simulink model "Exp9"  (R2018a)
settings: Solver=VariableStepAuto  StartTime=0.0  StopTime=0.2  RelTol=1e-3
libraries: powerlib x21
settings Model: Creator=Asus  LastModifiedBy=Asus

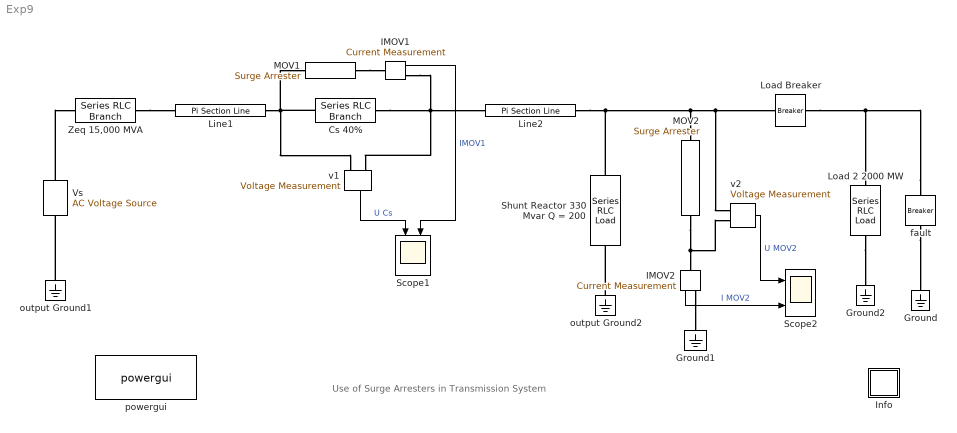
== system Exp9 ==
  note: Use of Surge Arresters in Transmission System
  Cs 40% : powerlib/Elements/Series RLC Branch  LConnTagsString=__new0  RConnTagsString=__new0  BranchType=C  Resistance=[]  Inductance=[]  SetiL0=off  InitialCurrent=0  Capacitance=101.4e-6  Setx0=off  InitialVoltage=0  Measurements=None
  Ground : powerlib/Elements/Ground  LConnTagsString=a
  Ground1 : powerlib/Elements/Ground  LConnTagsString=a
  Ground2 : powerlib/Elements/Ground  LConnTagsString=a
  IMOV1 : powerlib/Measurements/Current Measurement  Tag=PoWeRsYsTeMmEaSuReMeNt  PhasorSimulation=off  OutputType=Magnitude  PSBequivalent=0
  IMOV2 : powerlib/Measurements/Current Measurement  Tag=PoWeRsYsTeMmEaSuReMeNt  PhasorSimulation=off  OutputType=Magnitude  PSBequivalent=0
  Info : Subsystem
      settings: OpenFcn=showdemo(bdroot(gcb))
      mask Display: disp('?')
  Line1 : powerlib/Elements/Pi Section Line  LConnTagsString=__new0  RConnTagsString=__new0  Frequency=60  Resistance=0.011  Inductance=0.8674e-3  Capacitance=13.41e-9  Length=100  PiSections=2  Measurements=None
      settings: AttributesFormatString=\n  SourceProductName=Simscape Power Systems  SourceProductBaseCode=PS
  Line2 : powerlib/Elements/Pi Section Line  LConnTagsString=__new0  RConnTagsString=__new0  Frequency=60  Resistance=0.011  Inductance=0.8674e-3  Capacitance=13.41e-9  Length=100  PiSections=2  Measurements=None
      settings: AttributesFormatString=\n  SourceProductName=Simscape Power Systems  SourceProductBaseCode=PS
  Load 2 2000 MW : powerlib/Elements/Series RLC Load  LConnTagsString=a  RConnTagsString=__new0  NominalVoltage=735e3/sqrt(3)  NominalFrequency=60  ActivePower=2000e6/3  InductivePower=0  CapacitivePower=0  Setx0=off  InitialVoltage=0  SetiL0=off  InitialCurrent=0  Measurements=None  LoadType=constant Z
  Load Breaker : powerlib/Elements/Breaker  InitialState=1  SwitchingTimes=[ 100e-3]  External=off  BreakerResistance=0.1  SnubberResistance=inf  SnubberCapacitance=0  Measurements=None  MoreParameters=off  NoBreakLoop=off
      settings: AttributesFormatString=\n  SourceProductName=Simscape Power Systems
  MOV1 : powerlib/Elements/Surge Arrester  ProtectionVoltage=185e3  Columns=30  ReferenceCurrent=500  Segment1=[.955 50]  Segment2=[1.0 25]  Segment3=[.9915 16.5]  Measurements=None  BreakLoop=off
      settings: AttributesFormatString=\n  SourceProductName=Simscape Power Systems  SourceProductBaseCode=PS
  MOV2 : powerlib/Elements/Surge Arrester  ProtectionVoltage=1081e3  Columns=2  ReferenceCurrent=500  Segment1=[.955 50]  Segment2=[1.0 25]  Segment3=[.9915 16.5]  Measurements=None  BreakLoop=off
      settings: AttributesFormatString=\n  SourceProductName=Simscape Power Systems  SourceProductBaseCode=PS
  Scope1 : Scope  NumInputPorts=2
  Scope2 : Scope  NumInputPorts=2
  Shunt Reactor 330 Mvar Q = 200 : powerlib/Elements/Series RLC Load  LConnTagsString=a  RConnTagsString=__new0  NominalVoltage=735e3/sqrt(3)  NominalFrequency=60  ActivePower=330e6/3/200  InductivePower=330e6/3  CapacitivePower=0  Setx0=off  InitialVoltage=0  SetiL0=off  InitialCurrent=0  Measurements=None  LoadType=constant Z
  Vs : powerlib/Electrical Sources/AC Voltage Source  Description=source block  Amplitude=735e3/sqrt(3)*sqrt(2)  Phase=0  Frequency=60  SampleTime=0  Measurements=None  BusType=swing  Pref=10e3  Qref=0  Qmin=-inf  Qmax=+inf
      settings: AttributesFormatString=\n
  Zeq 15,000 MVA : powerlib/Elements/Series RLC Branch  LConnTagsString=__new0  RConnTagsString=__new0  BranchType=RL  Resistance=3.6  Inductance=95.5e-3  SetiL0=off  InitialCurrent=0  Capacitance=[]  Setx0=off  InitialVoltage=0  Measurements=None
  fault : powerlib/Elements/Breaker  InitialState=0  SwitchingTimes=[ 30e-3 300e-3]  External=off  BreakerResistance=1  SnubberResistance=inf  SnubberCapacitance=0  Measurements=None  MoreParameters=off  NoBreakLoop=off
      settings: AttributesFormatString=\n  SourceProductName=Simscape Power Systems
  output Ground1 : powerlib/Elements/Ground  LConnTagsString=a
  output Ground2 : powerlib/Elements/Ground  LConnTagsString=a
  powergui : powerlib/powergui  Priority=2  SimulationMode=Continuous  SampleTime=50e-6  frequency=60  Iterations=50  frequencyindice=60  Pbase=100e6  ErrMax=1e-4  UnitsV=kV  UnitsW=MW  buscounter=0  FunctionMessages=off  echomessages=off  EnableUseOfTLC=off  CurrentSourceSwitches=off  DisableSnubberDevices=off  DisableRonSwitches=off  DisableVfSwitches=off  DisplayEquations=off  SolverType=Tustin/Backward Euler (TBE)  Interpol=off  ExternalGateDelay=off  methode=off  Ts=100  x0status=blocks  SPID=on  SwTol=0  HookPort=off  RestoreLinks=warning  ResistiveCurrentMeasurement=off  Frange=logspace(0,3,50)  Ylog=off  Xlog=off  ShowGrid=off  save=off  variable=ZData  structure=0  ZoomFFT=on  StartTime=0.0  cycles=1  DisplayStyle=off  fundamental=60  FreqAxis=off  MaxFrequency=1000  frequencyindicesteady=1  RmsSteady=1  display=off
  v1 : powerlib/Measurements/Voltage Measurement  Tag=PoWeRsYsTeMmEaSuReMeNt  PhasorSimulation=off  OutputType=Magnitude  PSBequivalent=0
  v2 : powerlib/Measurements/Voltage Measurement  Tag=PoWeRsYsTeMmEaSuReMeNt  PhasorSimulation=off  OutputType=Magnitude  PSBequivalent=0
  wires:
  IMOV1/1 -> Scope1/2  "IMOV1"
  v1/1 -> Scope1/1  "U Cs"
  v2/1 -> Scope2/1  "U MOV2"
  IMOV2/1 -> Scope2/2  "I MOV2"
  connections:
  fault/LConn1 -- Load Breaker/RConn1 -- Load 2 2000 MW/LConn1
  v2/LConn1 -- Line2/RConn1 -- Shunt Reactor 330 Mvar Q = 200/RConn1 -- MOV2/LConn1 -- Load Breaker/LConn1
  v1/LConn2 -- Cs 40%/RConn1 -- Line2/LConn1 -- IMOV1/RConn1
  v2/LConn2 -- MOV2/RConn1 -- IMOV2/LConn1
  v1/LConn1 -- Cs 40%/LConn1 -- Line1/RConn1 -- MOV1/LConn1
  output Ground2/LConn1 -- Shunt Reactor 330 Mvar Q = 200/LConn1
  IMOV2/RConn1 -- Ground1/LConn1
  Vs/RConn1 -- Zeq 15,000 MVA/LConn1
  fault/RConn1 -- Ground/LConn1
  Load 2 2000 MW/RConn1 -- Ground2/LConn1
  Zeq 15,000 MVA/RConn1 -- Line1/LConn1
  MOV1/RConn1 -- IMOV1/LConn1
  output Ground1/LConn1 -- Vs/LConn1

== system Exp9/Info ==
